simulink model "hw9q4"  (R2018b)
settings: Solver=VariableStepAuto  StartTime=0.0  StopTime=100  RelTol=1e-6
settings Model: Creator=1  LastModifiedBy=1
settings SolverCC: ZeroCrossAlgorithm=Adaptive
settings DebuggingCC: IgnoredZcDiagnostic=none

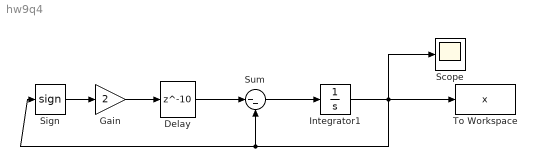
== system hw9q4 ==
  Delay : Delay  DelayLength=10  SampleTime=1
  Gain : Gain  Gain=2
  Integrator1 : Integrator  InitialCondition=10
  Scope : Scope
  Sign : Signum
  Sum : Sum  Inputs=|--
  To Workspace : ToWorkspace  VariableName=x  SaveFormat=Timeseries  SampleTime=-1
  wires:
  Sum/1 -> Integrator1/1
  Integrator1/1 -> Sign/1, Sum/2, To Workspace/1, Scope/1
  Sign/1 -> Gain/1
  Gain/1 -> Delay/1
  Delay/1 -> Sum/1
